simulink model "swinging_pendulum"  (R2023b)
settings: Solver=VariableStepAuto  StartTime=0.0  StopTime=20  RelTol=1e-3
values from neighbouring files (symbols this model uses):
  alpha_0 = cutData(1)    [model_validation_data.m]    (also in pendulum_experiment.m)
  Bp_ = 1.51e-5    (= 1.51e-05)    [model_validation_data.m]    (also in pendulum_experiment.m = 1e-06)
  g_ = 9.81    [model_validation_data.m]    (also in pendulum_experiment.m)
  Jp_ = 2.44e-5    (= 2.44e-05)    [model_validation_data.m]    (also in pendulum_experiment.m = 3.342606e-05)
  lp_ = Lp/2    (= 0.0645)    [model_validation_data.m]    (also in pendulum_experiment.m)
  mp_ = 0.024    [model_validation_data.m]    (also in pendulum_experiment.m)
settings Model: Creator=renzo  LastModifiedBy=renzo
settings DataIOCC: SaveFormat=StructureWithTime

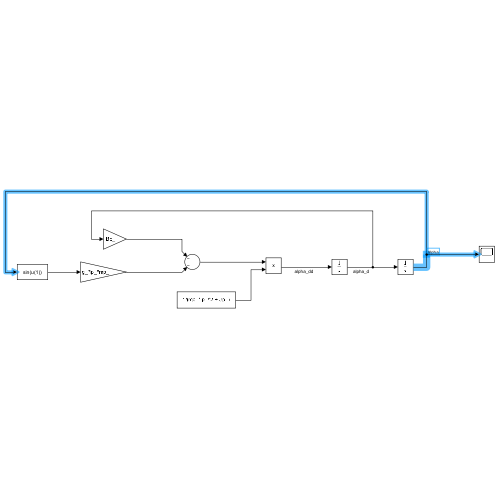
[thumbnail: Simulink's stored preview of the top-level diagram]
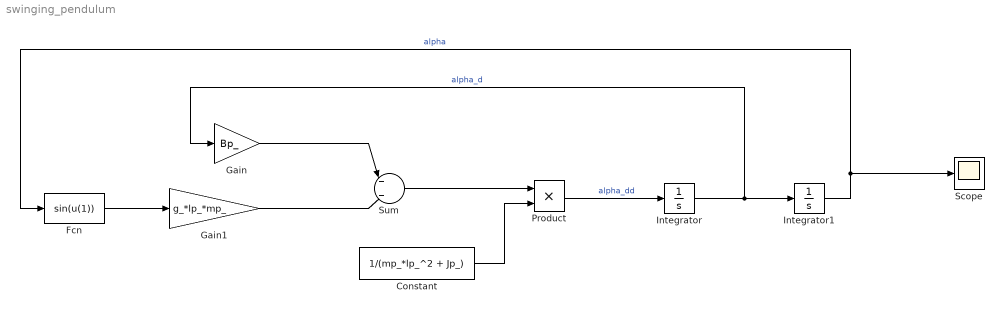
== system swinging_pendulum ==
  Constant : Constant  Value=1/(mp_*lp_^2 + Jp_)
  Fcn : Fcn  Expr=sin(u(1))
  Gain : Gain  Gain=Bp_
  Gain1 : Gain  Gain=g_*lp_*mp_
  Integrator : Integrator
  Integrator1 : Integrator  InitialCondition=alpha_0
  Product : Product
  Scope : Scope
  Sum : Sum  Inputs=|-|-|
  wires:
  Product/1 -> Integrator/1  "alpha_dd"
  Integrator/1 -> Gain/1, Integrator1/1  "alpha_d"
  Constant/1 -> Product/2
  Sum/1 -> Product/1
  Gain/1 -> Sum/1
  Gain1/1 -> Sum/2
  Fcn/1 -> Gain1/1
  Integrator1/1 -> Scope/1, Fcn/1  "alpha"
